simulink model "RLC_simulink"  (R2015a)
settings: Solver=ode8  StartTime=0.0  StopTime=500  FixedStep=0.0001  RelTol=1e-3
undefined symbols (not defined in the file or in its folder): C, L, R
settings Model: Creator=DELL  LastModifiedBy=DELL

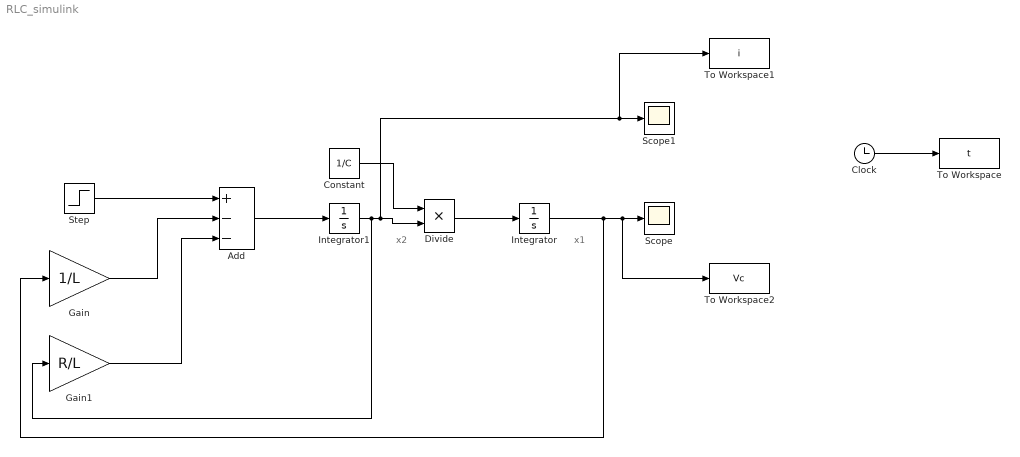
== system RLC_simulink ==
  note: x1
  note: x2
  Add : Sum  Inputs=+--
  Clock : Clock
  Constant : Constant  Value=1/C
  Divide : Product  Inputs=**
  Gain : Gain  Gain=1/L
  Gain1 : Gain  Gain=R/L
  Integrator : Integrator
  Integrator1 : Integrator
  Scope : Scope
  Scope1 : Scope
  Step : Step  Time=0  After=e/L  SampleTime=0
  To Workspace : ToWorkspace  VariableName=t  SampleTime=-1
  To Workspace1 : ToWorkspace  VariableName=i  SampleTime=-1
  To Workspace2 : ToWorkspace  VariableName=Vc  SampleTime=-1
  wires:
  Add/1 -> Integrator1/1
  Step/1 -> Add/1
  Gain/1 -> Add/2
  Gain1/1 -> Add/3
  Integrator1/1 -> Gain1/1, To Workspace1/1, Scope1/1, Divide/2
  Constant/1 -> Divide/1
  Divide/1 -> Integrator/1
  Integrator/1 -> To Workspace2/1, Scope/1, Gain/1
  Clock/1 -> To Workspace/1
